simulink model "Pure Least Squares with Covariance Resetting"  (R2020a)
settings: Solver=VariableStepAuto  StartTime=0.0  StopTime=250  RelTol=1e-13  AbsTol=1e-9
InitFcn:
  | r0=10;
  | theta_est1=[3; 1.5];
  | theta_est2=[1;2];
  | r1=1;
undefined symbols (not defined in the file): theta_ref1, theta_ref2
libraries: dspinverses x1, dspfactors x1
settings Model: Creator=Haris  LastModifiedBy=Haris

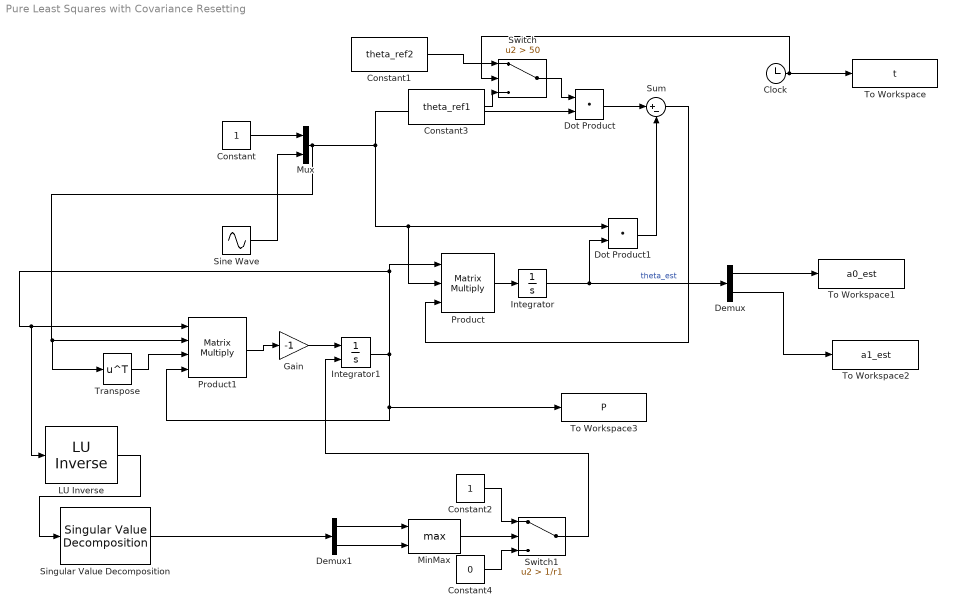
== system Pure Least Squares with Covariance Resetting ==
  " LU Inverse" : dspinverses/ LU Inverse
  Clock : Clock
  Constant : Constant
  Constant1 : Constant  Value=theta_ref2
  Constant2 : Constant
  Constant3 : Constant  Value=theta_ref1
  Constant4 : Constant  Value=0
  Demux : Demux  Outputs=2
  Demux1 : Demux  Outputs=2
  Dot Product : DotProduct  InputSameDT=on  OutDataTypeStr=Inherit: Inherit via internal rule
  Dot Product1 : DotProduct  InputSameDT=on  OutDataTypeStr=Inherit: Inherit via internal rule
  Gain : Gain  Gain=-1
  Integrator : Integrator  InitialCondition=[0;0]
  Integrator1 : Integrator  ExternalReset=rising  InitialCondition=diag([r0 r0])
  MinMax : MinMax  Function=max  Inputs=2
  Mux : Mux  Inputs=2
  Product : Product  Inputs=3  Multiplication=Matrix(*)
  Product1 : Product  Inputs=4  Multiplication=Matrix(*)
  Sine Wave : Sin  SampleTime=0
  Singular Value Decomposition : dspfactors/Singular Value Decomposition  wantv=on  wanterr=off  SimulateUsing=Interpreted execution
      settings: SourceProductBaseCode=DS
  Sum : Sum  Inputs=|+-
  Switch : Switch  Criteria=u2 > Threshold  Threshold=50
  Switch1 : Switch  Criteria=u2 > Threshold  Threshold=1/r1
  To Workspace : ToWorkspace  VariableName=t  SampleTime=-1
  To Workspace1 : ToWorkspace  VariableName=a0_est  SampleTime=-1
  To Workspace2 : ToWorkspace  VariableName=a1_est  SampleTime=-1
  To Workspace3 : ToWorkspace  VariableName=P  SampleTime=-1
  Transpose : Math  Operator=transpose  SaturateOnIntegerOverflow=on
  wires:
  Constant/1 -> Mux/1
  Sine Wave/1 -> Mux/2
  Mux/1 -> Transpose/1, Product1/2, Product/2, Dot Product1/1, Dot Product/2
  Dot Product/1 -> Sum/1
  Dot Product1/1 -> Sum/2
  Integrator/1 -> Demux/1, Dot Product1/2  "theta_est"
  Product/1 -> Integrator/1
  Integrator1/1 -> " LU Inverse"/1, Product1/1, Product/1, To Workspace3/1, Product1/4
  Sum/1 -> Product/3
  Gain/1 -> Integrator1/1
  Product1/1 -> Gain/1
  Transpose/1 -> Product1/3
  Switch1/1 -> Integrator1/2
  Clock/1 -> Switch/2, To Workspace/1
  Demux/1 -> To Workspace1/1
  Demux/2 -> To Workspace2/1
  Constant1/1 -> Switch/1
  Constant3/1 -> Switch/3
  Switch/1 -> Dot Product/1
  " LU Inverse"/1 -> Singular Value Decomposition/1
  MinMax/1 -> Switch1/2
  Singular Value Decomposition/2 -> Demux1/1
  Demux1/1 -> MinMax/1
  Demux1/2 -> MinMax/2
  Constant2/1 -> Switch1/1
  Constant4/1 -> Switch1/3
